simulink model "gpc_siso_delay_1_sim"  (R2022a)
settings: Solver=VariableStepAuto  StartTime=0.0  StopTime=Tsim  RelTol=1e-3
values from neighbouring files (symbols this model uses):
  A = A'    [gpc_siso_delay_1.m]
  B = B'    [gpc_siso_delay_1.m]
  D = D'    [gpc_siso_delay_1.m]
  delta = 1    [gpc_siso_delay_1.m]
  F = cell2mat(F)    [gpc_siso_delay_1.m]
  H = H'    [gpc_siso_delay_1.m]
  K = Aux(size(B,2),:)    [gpc_siso_delay_1.m]
  Kr = sum(K)    [gpc_siso_delay_1.m]
  Ld = ceil(L/Ts)    [gpc_siso_delay_1.m]
  Ts = 1    [gpc_siso_delay_1.m]
libraries: cstblocks x2
settings Model: Creator=aaron  LastModifiedBy=aaron

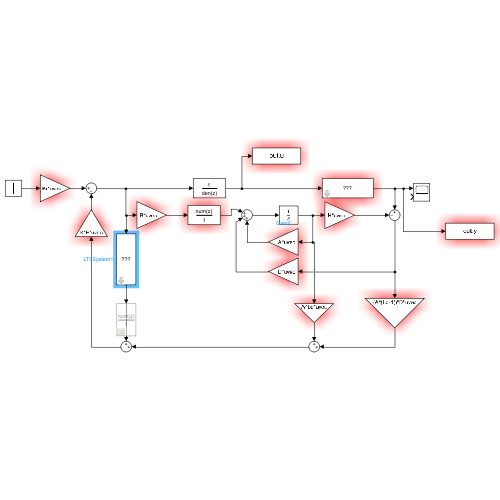
[thumbnail: Simulink's stored preview of the top-level diagram]
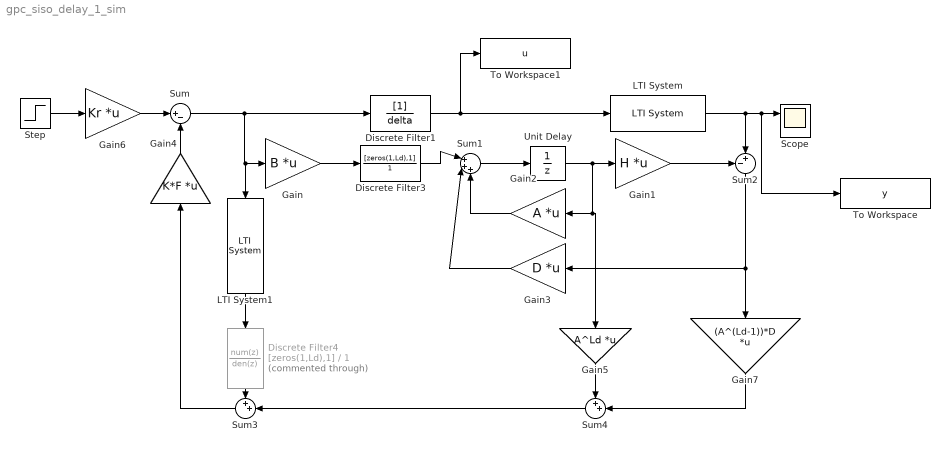
== system gpc_siso_delay_1_sim ==
  Discrete Filter1 : DiscreteFilter  Denominator=delta
  Discrete Filter3 : DiscreteFilter  Numerator=[zeros(1,Ld),1]  Denominator=1
  Discrete Filter4 : DiscreteFilter  Commented=through  Numerator=[zeros(1,Ld),1]  Denominator=1
  Gain : Gain  Gain=B  Multiplication=Matrix(K*u) (u vector)
  Gain1 : Gain  Gain=H  Multiplication=Matrix(K*u) (u vector)
  Gain2 : Gain  Gain=A  Multiplication=Matrix(K*u) (u vector)
  Gain3 : Gain  Gain=D  Multiplication=Matrix(K*u) (u vector)
  Gain4 : Gain  Gain=K*F  Multiplication=Matrix(K*u) (u vector)
  Gain5 : Gain  Gain=A^Ld  Multiplication=Matrix(K*u) (u vector)
  Gain6 : Gain  Gain=Kr  Multiplication=Matrix(K*u) (u vector)
  Gain7 : Gain  Gain=(A^(Ld-1))*D  Multiplication=Matrix(K*u) (u vector)
  LTI System : cstblocks/LTI System  sys=P  IC=[]
  LTI System1 : cstblocks/LTI System  sys=Ftil  IC=[]
  Scope : Scope  NumInputPorts=2
  Step : Step  Time=0  SampleTime=0
  Sum : Sum  Inputs=|+-
  Sum1 : Sum  Inputs=|+++
  Sum2 : Sum  Inputs=-+|
  Sum3 : Sum  Inputs=++|
  Sum4 : Sum  Inputs=++|
  To Workspace : ToWorkspace  VariableName=y  SampleTime=Ts
  To Workspace1 : ToWorkspace  VariableName=u  SampleTime=Ts
  Unit Delay : UnitDelay  SampleTime=-1  HasFrameUpgradeWarning=on
  wires:
  Gain6/1 -> Sum/1
  Step/1 -> Gain6/1
  Sum1/1 -> Unit Delay/1
  Gain1/1 -> Sum2/1
  LTI System/1 -> To Workspace/1, Scope/1, Sum2/2
  Discrete Filter1/1 -> To Workspace1/1, LTI System/1
  Sum/1 -> Discrete Filter1/1, LTI System1/1, Gain/1
  Unit Delay/1 -> Gain2/1, Gain5/1, Gain1/1
  Gain2/1 -> Sum1/3
  Sum2/1 -> Gain3/1, Gain7/1
  Gain3/1 -> Sum1/2
  Gain4/1 -> Sum/2
  Sum3/1 -> Gain4/1
  Gain5/1 -> Sum4/1
  Gain7/1 -> Sum4/2
  Sum4/1 -> Sum3/2
  Discrete Filter3/1 -> Sum1/1
  Gain/1 -> Discrete Filter3/1
  LTI System1/1 -> Discrete Filter4/1
  Discrete Filter4/1 -> Sum3/1
